simulink model "attitude_kalman_filter"  (R2023a)
settings: configuration reference "configuration_filter" (kept outside this file)
undefined symbols (not defined in the file): correction_performed_bool, Eul_rad, filt, rot_K_est_bias_OB_B_radDs, rot_K_est_OB_B_radDs, sfor_est_B_mDs, sfor_est_bias_B_mDs2
libraries: lib_jacobians x5, lib_kinematics x1
settings Model: Creator=FC_dev1  LastModifiedBy=FC_dev1
settings ConfigSetRef: SourceName=configuration_filter  SourceLocation=Base Workspace

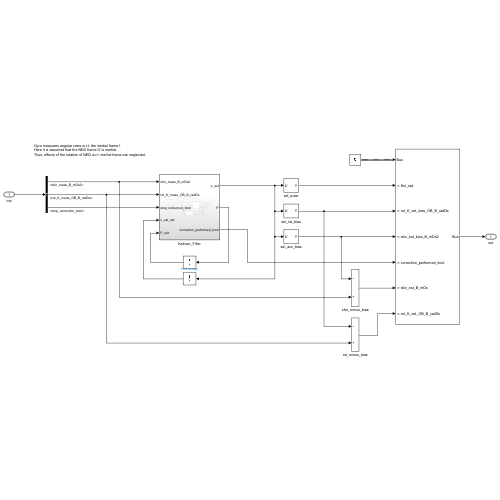
[thumbnail: Simulink's stored preview of the top-level diagram]
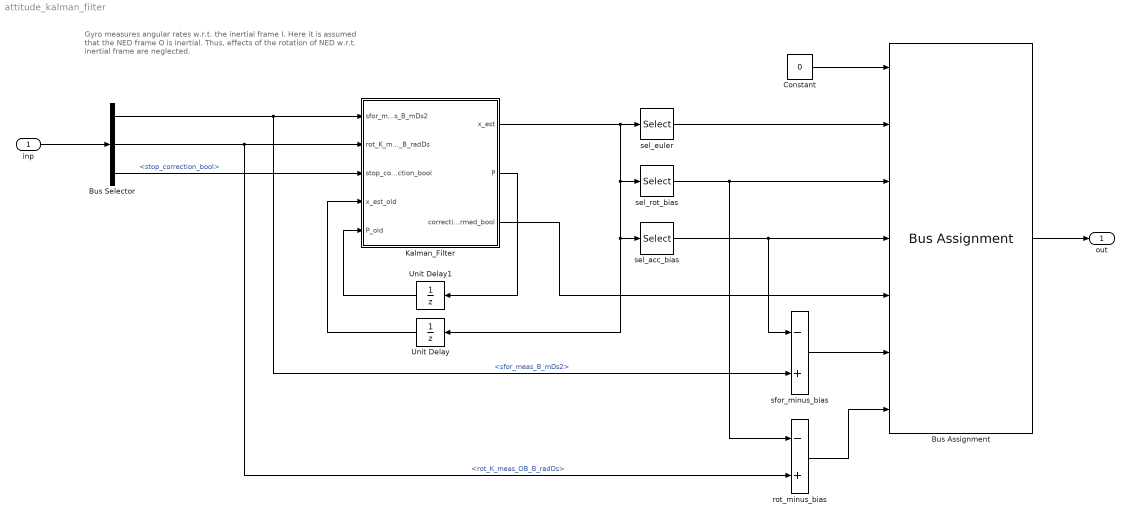
== system attitude_kalman_filter ==
  note: Gyro measures angular rates w.r.t. the inertial frame I.
      | Here it is assumed that the NED frame O is inertial.
      | Thus, effects of the rotation of NED w.r.t. inertial frame are neglected.
  inp : Inport  OutDataTypeStr=Bus: inp_Bus
  Bus Assignment : BusAssignment  AssignedSignals=Eul_rad,rot_K_est_bias_OB_B_radDs,sfor_est_bias_B_mDs2,correction_performed_bool,sfor_est_B_mDs,rot_K_est_OB_B_radDs
  Bus Selector : BusSelector  OutputSignals=sfor_meas_B_mDs2,rot_K_meas_OB_B_radDs,stop_correction_bool
  Constant : Constant  Value=0  OutDataTypeStr=Bus: out_Bus
  Kalman_Filter : Subsystem
  Unit Delay : UnitDelay  InitialCondition=filt.x0  SampleTime=-1  HasFrameUpgradeWarning=on
  Unit Delay1 : UnitDelay  InitialCondition=filt.P0  SampleTime=-1  HasFrameUpgradeWarning=on
  rot_minus_bias : Sum  Inputs=-+
  sel_acc_bias : Selector  NumberOfDimensions=2  InputPortWidth=3  IndexOptions=Index vector (dialog),Index vector (dialog)  Indices=filt.acc_bias_idx,1  OutputSizes=1,1
  sel_euler : Selector  NumberOfDimensions=2  InputPortWidth=3  IndexOptions=Index vector (dialog),Index vector (dialog)  Indices=filt.eul_idx,1  OutputSizes=1,1
  sel_rot_bias : Selector  NumberOfDimensions=2  InputPortWidth=3  IndexOptions=Index vector (dialog),Index vector (dialog)  Indices=filt.rot_bias_idx,1  OutputSizes=1,1
  sfor_minus_bias : Sum  Inputs=-+
  out : Outport  OutDataTypeStr=Bus: out_Bus
  wires:
  sel_euler/1 -> Bus Assignment/2
  Kalman_Filter/2(P) -> Unit Delay1/1
  Bus Selector/1 -> sfor_minus_bias/2, Kalman_Filter/1(sfor_meas_B_mDs2)  "<sfor_meas_B_mDs2>"
  Bus Selector/2 -> rot_minus_bias/2, Kalman_Filter/2(rot_K_meas_OB_B_radDs)  "<rot_K_meas_OB_B_radDs>"
  Unit Delay1/1 -> Kalman_Filter/5(P_old)
  Unit Delay/1 -> Kalman_Filter/4(x_est_old)
  Bus Selector/3 -> Kalman_Filter/3(stop_correction_bool)  "<stop_correction_bool>"
  Kalman_Filter/1(x_est) -> sel_rot_bias/1, Unit Delay/1, sel_acc_bias/1, sel_euler/1
  sel_rot_bias/1 -> Bus Assignment/3, rot_minus_bias/1
  sel_acc_bias/1 -> sfor_minus_bias/1, Bus Assignment/4
  Kalman_Filter/3(correction_performed_bool) -> Bus Assignment/5
  sfor_minus_bias/1 -> Bus Assignment/6
  rot_minus_bias/1 -> Bus Assignment/7
  Constant/1 -> Bus Assignment/1
  Bus Assignment/1 -> out/1
  inp/1 -> Bus Selector/1

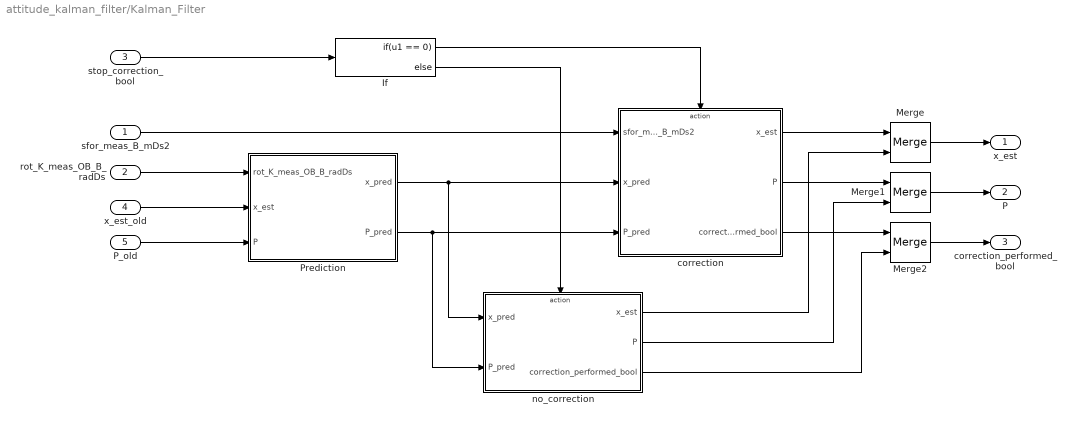
== system attitude_kalman_filter/Kalman_Filter ==
  sfor_meas_B_mDs2 : Inport
  rot_K_meas_OB_B_radDs : Inport  Port=2
  stop_correction_bool : Inport  Port=3
  x_est_old : Inport  Port=4
  P_old : Inport  Port=5
  If : If  IfExpression=u1 == 0
  Merge : Merge
  Merge1 : Merge
  Merge2 : Merge
  Prediction : Subsystem
  correction : Subsystem
  no_correction : Subsystem
  x_est : Outport
  P : Outport  Port=2
  correction_performed_bool : Outport  Port=3
  wires:
  Prediction/2(P_pred) -> correction/3(P_pred), no_correction/2(P_pred)
  x_est_old/1 -> Prediction/2(x_est)
  correction/2(P) -> Merge1/1
  sfor_meas_B_mDs2/1 -> correction/1(sfor_meas_B_mDs2)
  Prediction/1(x_pred) -> correction/2(x_pred), no_correction/1(x_pred)
  rot_K_meas_OB_B_radDs/1 -> Prediction/1(rot_K_meas_OB_B_radDs)
  correction/1(x_est) -> Merge/1
  P_old/1 -> Prediction/3(P)
  stop_correction_bool/1 -> If/1
  If/1 -> correction/Action
  Merge/1 -> x_est/1
  Merge1/1 -> P/1
  If/2 -> no_correction/Action
  no_correction/1(x_est) -> Merge/2
  no_correction/2(P) -> Merge1/2
  Merge2/1 -> correction_performed_bool/1
  correction/3(correction_performed_bool) -> Merge2/1
  no_correction/3(correction_performed_bool) -> Merge2/2

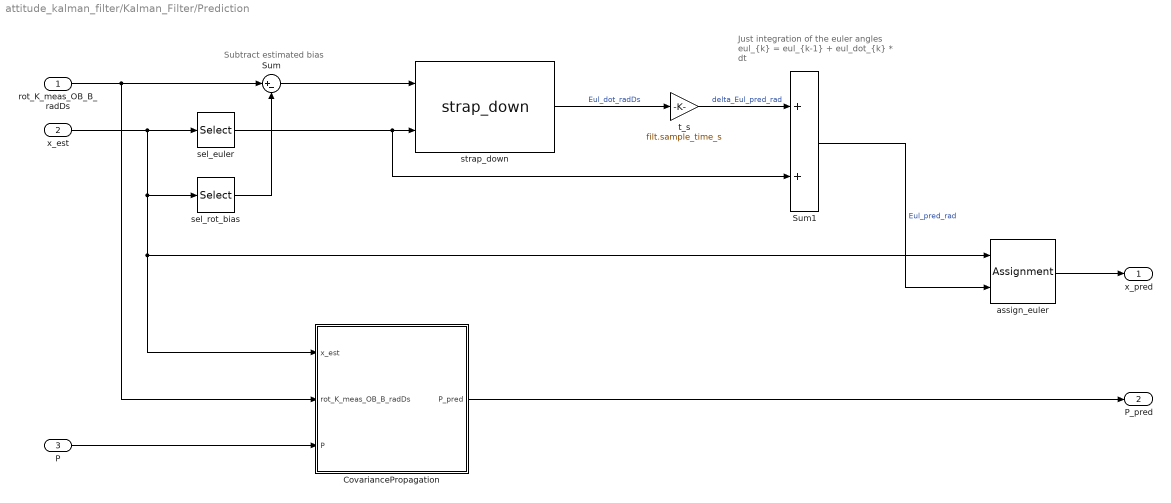
== system attitude_kalman_filter/Kalman_Filter/Prediction ==
  note: Just integration of the euler angles
      | eul_{k} = eul_{k-1} + eul_dot_{k} * dt
  note: Subtract estimated bias
  rot_K_meas_OB_B_radDs : Inport
  x_est : Inport  Port=2
  P : Inport  Port=3
  CovariancePropagation : Subsystem
  Sum : Sum  Inputs=|+-
  Sum1 : Sum
  assign_euler : Assignment  NumberOfDimensions=2  DiagnosticForDimensions=Warning  IndexOptions=Index vector (dialog),Index vector (dialog)  Indices=filt.eul_idx,1  OutputSizes=1,1
  sel_euler : Selector  NumberOfDimensions=2  InputPortWidth=3  IndexOptions=Index vector (dialog),Index vector (dialog)  Indices=filt.eul_idx,1  OutputSizes=1,1
  sel_rot_bias : Selector  NumberOfDimensions=2  InputPortWidth=3  IndexOptions=Index vector (dialog),Index vector (dialog)  Indices=filt.rot_bias_idx,1  OutputSizes=1,1
  strap_down : lib_kinematics/strap_down  SystemSampleTime=-1  VariantActivationTime=update diagram  Latency=0  AutoFrameSizeCalculation=off
  t_s : Gain  Gain=filt.sample_time_s
  x_pred : Outport
  P_pred : Outport  Port=2
  wires:
  rot_K_meas_OB_B_radDs/1 -> CovariancePropagation/2(rot_K_meas_OB_B_radDs), Sum/1
  x_est/1 -> CovariancePropagation/1(x_est), assign_euler/1, sel_rot_bias/1, sel_euler/1
  P/1 -> CovariancePropagation/3(P)
  CovariancePropagation/1(P_pred) -> P_pred/1
  sel_euler/1 -> Sum1/2, strap_down/2
  Sum/1 -> strap_down/1
  sel_rot_bias/1 -> Sum/2
  strap_down/1 -> t_s/1  "Eul_dot_radDs"
  t_s/1 -> Sum1/1  "delta_Eul_pred_rad"
  Sum1/1 -> assign_euler/2  "Eul_pred_rad"
  assign_euler/1 -> x_pred/1

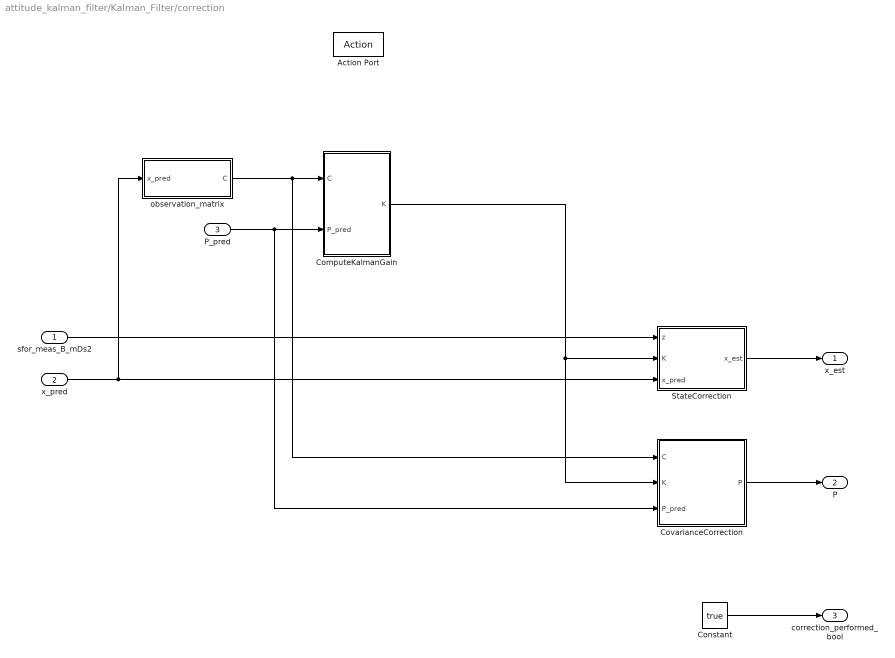
== system attitude_kalman_filter/Kalman_Filter/correction ==
  sfor_meas_B_mDs2 : Inport
  x_pred : Inport  Port=2
  P_pred : Inport  Port=3
  Action Port : ActionPort  ActionPortLabel=if(u1 == 0)
  ComputeKalmanGain : Subsystem
  Constant : Constant  Value=true
  CovarianceCorrection : Subsystem
  StateCorrection : Subsystem
  observation_matrix : Subsystem
  x_est : Outport
  P : Outport  Port=2
  correction_performed_bool : Outport  Port=3
  wires:
  P_pred/1 -> CovarianceCorrection/3(P_pred), ComputeKalmanGain/2(P_pred)
  observation_matrix/1(C) -> CovarianceCorrection/1(C), ComputeKalmanGain/1(C)
  StateCorrection/1(x_est) -> x_est/1
  CovarianceCorrection/1(P) -> P/1
  x_pred/1 -> observation_matrix/1(x_pred), StateCorrection/3(x_pred)
  ComputeKalmanGain/1(K) -> CovarianceCorrection/2(K), StateCorrection/2(K)
  sfor_meas_B_mDs2/1 -> StateCorrection/1(z)
  Constant/1 -> correction_performed_bool/1

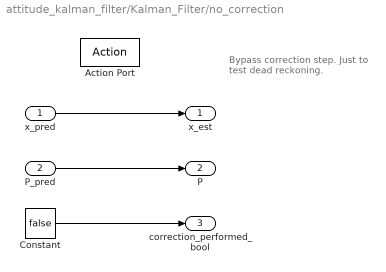
== system attitude_kalman_filter/Kalman_Filter/no_correction ==
  note: Bypass correction step.
      | Just to test dead reckoning.
  x_pred : Inport
  P_pred : Inport  Port=2
  Action Port : ActionPort  ActionPortLabel=else
  Constant : Constant  Value=false
  x_est : Outport
  P : Outport  Port=2
  correction_performed_bool : Outport  Port=3
  wires:
  P_pred/1 -> P/1
  x_pred/1 -> x_est/1
  Constant/1 -> correction_performed_bool/1

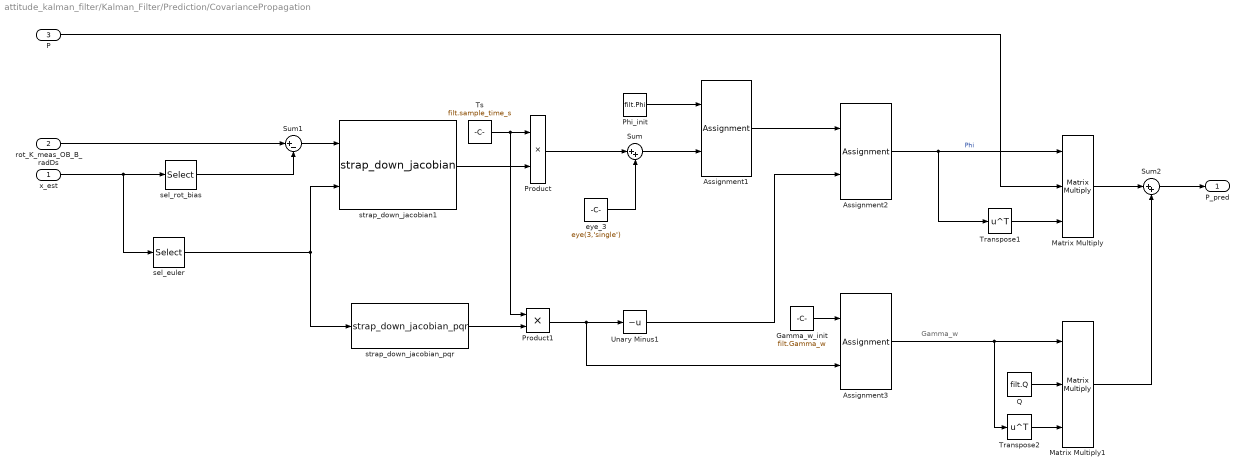
== system attitude_kalman_filter/Kalman_Filter/Prediction/CovariancePropagation ==
  note: Gamma_w
  x_est : Inport
  rot_K_meas_OB_B_radDs : Inport  Port=2
  P : Inport  Port=3
  Assignment1 : Assignment  NumberOfDimensions=2  DiagnosticForDimensions=Warning  IndexOptions=Index vector (dialog),Index vector (dialog)  Indices=filt.eul_idx,filt.eul_idx  OutputSizes=1,1
  Assignment2 : Assignment  NumberOfDimensions=2  DiagnosticForDimensions=Warning  IndexOptions=Index vector (dialog),Index vector (dialog)  Indices=filt.rot_bias_idx,filt.rot_bias_idx  OutputSizes=1,1
  Assignment3 : Assignment  NumberOfDimensions=2  DiagnosticForDimensions=Warning  IndexOptions=Index vector (dialog),Index vector (dialog)  Indices=filt.eul_idx,filt.rot_noise_idx  OutputSizes=1,1
  Gamma_w_init : Constant  Value=filt.Gamma_w  VectorParams1D=off
  Matrix Multiply : Product  Inputs=3  Multiplication=Matrix(*)
  Matrix Multiply1 : Product  Inputs=3  Multiplication=Matrix(*)
  Phi_init : Constant  Value=filt.Phi  VectorParams1D=off
  Product : Product
  Product1 : Product
  Q : Constant  Value=filt.Q  VectorParams1D=off
  Sum : Sum  Inputs=|++
  Sum1 : Sum  Inputs=|+-
  Sum2 : Sum  Inputs=|++
  Transpose1 : Math  Operator=transpose
  Transpose2 : Math  Operator=transpose
  Ts : Constant  Value=filt.sample_time_s
  Unary Minus1 : UnaryMinus
  eye_3 : Constant  Value=eye(3,'single')  VectorParams1D=off
  sel_euler : Selector  NumberOfDimensions=2  InputPortWidth=3  IndexOptions=Index vector (dialog),Index vector (dialog)  Indices=filt.eul_idx,1  OutputSizes=1,1
  sel_rot_bias : Selector  NumberOfDimensions=2  InputPortWidth=3  IndexOptions=Index vector (dialog),Index vector (dialog)  Indices=filt.rot_bias_idx,1  OutputSizes=1,1
  strap_down_jacobian1 : lib_jacobians/strap_down_jacobian  SystemSampleTime=-1  VariantActivationTime=update diagram  Latency=0  AutoFrameSizeCalculation=off
  strap_down_jacobian_pqr : lib_jacobians/strap_down_jacobian_pqr  SystemSampleTime=-1  VariantActivationTime=update diagram  Latency=0  AutoFrameSizeCalculation=off
  P_pred : Outport
  wires:
  P/1 -> Matrix Multiply/2
  Transpose1/1 -> Matrix Multiply/3
  x_est/1 -> sel_rot_bias/1, sel_euler/1
  sel_euler/1 -> strap_down_jacobian1/2, strap_down_jacobian_pqr/1
  rot_K_meas_OB_B_radDs/1 -> Sum1/1
  sel_rot_bias/1 -> Sum1/2
  strap_down_jacobian1/1 -> Product/2
  Product/1 -> Sum/1
  Phi_init/1 -> Assignment1/1
  Sum/1 -> Assignment1/2
  eye_3/1 -> Sum/2
  strap_down_jacobian_pqr/1 -> Product1/2
  Sum1/1 -> strap_down_jacobian1/1
  Product1/1 -> Unary Minus1/1, Assignment3/2
  Assignment1/1 -> Assignment2/1
  Unary Minus1/1 -> Assignment2/2
  Gamma_w_init/1 -> Assignment3/1
  Assignment2/1 -> Matrix Multiply/1, Transpose1/1  "Phi"
  Assignment3/1 -> Transpose2/1, Matrix Multiply1/1
  Transpose2/1 -> Matrix Multiply1/3
  Q/1 -> Matrix Multiply1/2
  Matrix Multiply/1 -> Sum2/1
  Sum2/1 -> P_pred/1
  Matrix Multiply1/1 -> Sum2/2
  Ts/1 -> Product1/1, Product/1

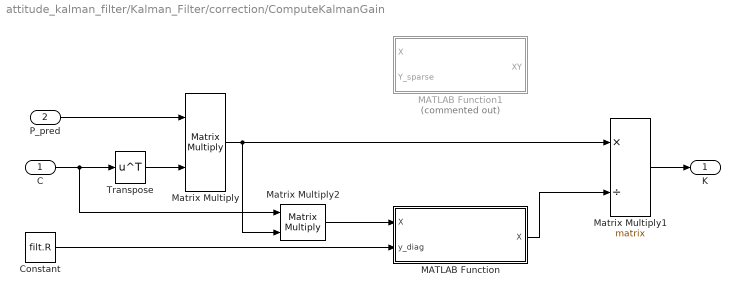
== system attitude_kalman_filter/Kalman_Filter/correction/ComputeKalmanGain ==
  C : Inport
  P_pred : Inport  Port=2
  Constant : Constant  Value=filt.R
  MATLAB Function : MATLAB Function  TreatAsAtomicUnit=on
  MATLAB Function1 : MATLAB Function  Commented=on  TreatAsAtomicUnit=on
  Matrix Multiply : Product  Multiplication=Matrix(*)
  Matrix Multiply1 : Product  Inputs=*/  Multiplication=Matrix(*)
  Matrix Multiply2 : Product  Multiplication=Matrix(*)
  Transpose : Math  Operator=transpose
  K : Outport
  wires:
  P_pred/1 -> Matrix Multiply/1
  Matrix Multiply/1 -> Matrix Multiply1/1, Matrix Multiply2/2
  C/1 -> Matrix Multiply2/1, Transpose/1
  Transpose/1 -> Matrix Multiply/2
  Matrix Multiply2/1 -> MATLAB Function/1("X ")
  MATLAB Function/1(X) -> Matrix Multiply1/2
  Constant/1 -> MATLAB Function/2(y_diag)
  Matrix Multiply1/1 -> K/1

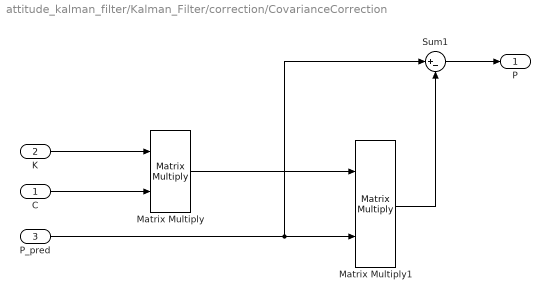
== system attitude_kalman_filter/Kalman_Filter/correction/CovarianceCorrection ==
  C : Inport
  K : Inport  Port=2
  P_pred : Inport  Port=3
  Matrix Multiply : Product  Multiplication=Matrix(*)
  Matrix Multiply1 : Product  Multiplication=Matrix(*)
  Sum1 : Sum  Inputs=|+-
  P : Outport
  wires:
  C/1 -> Matrix Multiply/2
  K/1 -> Matrix Multiply/1
  Matrix Multiply/1 -> Matrix Multiply1/1
  Matrix Multiply1/1 -> Sum1/2
  P_pred/1 -> Sum1/1, Matrix Multiply1/2
  Sum1/1 -> P/1

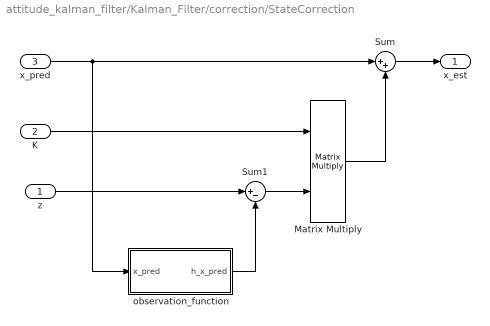
== system attitude_kalman_filter/Kalman_Filter/correction/StateCorrection ==
  z : Inport
  K : Inport  Port=2
  x_pred : Inport  Port=3
  Matrix Multiply : Product  Multiplication=Matrix(*)
  Sum : Sum  Inputs=|++
  Sum1 : Sum  Inputs=|+-
  observation_function : Subsystem
  x_est : Outport
  wires:
  x_pred/1 -> observation_function/1(x_pred), Sum/1
  K/1 -> Matrix Multiply/1
  Matrix Multiply/1 -> Sum/2
  Sum/1 -> x_est/1
  z/1 -> Sum1/1
  observation_function/1(h_x_pred) -> Sum1/2
  Sum1/1 -> Matrix Multiply/2

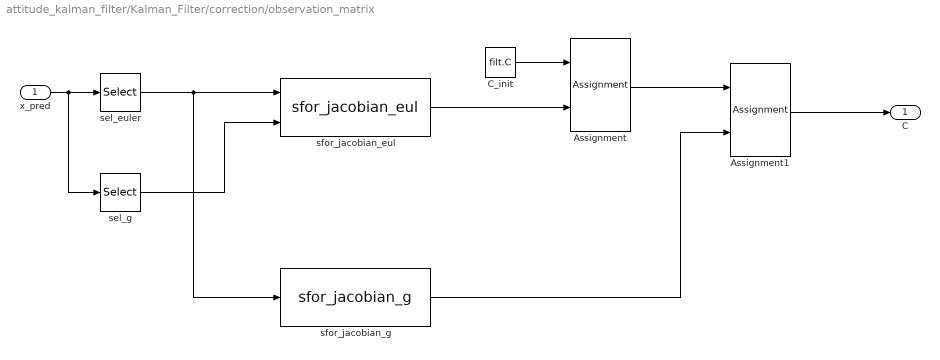
== system attitude_kalman_filter/Kalman_Filter/correction/observation_matrix ==
  x_pred : Inport
  Assignment : Assignment  NumberOfDimensions=2  DiagnosticForDimensions=Warning  IndexOptions=Assign all,Index vector (dialog)  Indices=1,filt.eul_idx  OutputSizes=1,1
  Assignment1 : Assignment  NumberOfDimensions=2  DiagnosticForDimensions=Warning  IndexOptions=Assign all,Index vector (dialog)  Indices=1,filt.g_idx  OutputSizes=1,1
  C_init : Constant  Value=filt.C  VectorParams1D=off
  sel_euler : Selector  NumberOfDimensions=2  InputPortWidth=3  IndexOptions=Index vector (dialog),Index vector (dialog)  Indices=filt.eul_idx,1  OutputSizes=1,1
  sel_g : Selector  NumberOfDimensions=2  InputPortWidth=3  IndexOptions=Index vector (dialog),Index vector (dialog)  Indices=filt.g_idx,1  OutputSizes=1,1
  sfor_jacobian_eul : lib_jacobians/sfor_jacobian_eul  SystemSampleTime=-1  VariantActivationTime=update diagram  Latency=0  AutoFrameSizeCalculation=off
  sfor_jacobian_g : lib_jacobians/sfor_jacobian_g  SystemSampleTime=-1  VariantActivationTime=update diagram  Latency=0  AutoFrameSizeCalculation=off
  C : Outport
  wires:
  x_pred/1 -> sel_g/1, sel_euler/1
  sel_euler/1 -> sfor_jacobian_eul/1, sfor_jacobian_g/1
  sel_g/1 -> sfor_jacobian_eul/2
  C_init/1 -> Assignment/1
  sfor_jacobian_eul/1 -> Assignment/2
  Assignment/1 -> Assignment1/1
  Assignment1/1 -> C/1
  sfor_jacobian_g/1 -> Assignment1/2

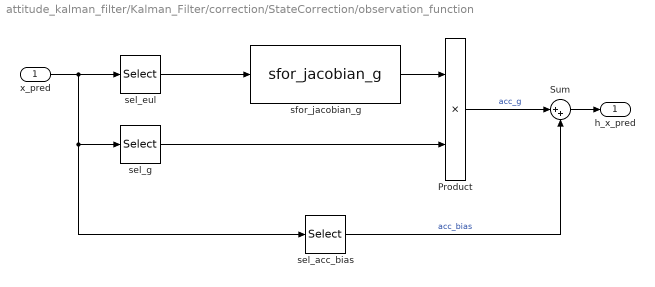
== system attitude_kalman_filter/Kalman_Filter/correction/StateCorrection/observation_function ==
  x_pred : Inport
  Product : Product
  Sum : Sum  Inputs=|++
  sel_acc_bias : Selector  NumberOfDimensions=2  InputPortWidth=3  IndexOptions=Index vector (dialog),Index vector (dialog)  Indices=filt.acc_bias_idx,1  OutputSizes=1,1
  sel_eul : Selector  NumberOfDimensions=2  InputPortWidth=3  IndexOptions=Index vector (dialog),Index vector (dialog)  Indices=filt.eul_idx,1  OutputSizes=1,1
  sel_g : Selector  NumberOfDimensions=2  InputPortWidth=3  IndexOptions=Index vector (dialog),Index vector (dialog)  Indices=filt.g_idx,1  OutputSizes=1,1
  sfor_jacobian_g : lib_jacobians/sfor_jacobian_g  SystemSampleTime=-1  VariantActivationTime=update diagram  Latency=0  AutoFrameSizeCalculation=off
  h_x_pred : Outport
  wires:
  x_pred/1 -> sel_acc_bias/1, sel_g/1, sel_eul/1
  Sum/1 -> h_x_pred/1
  sel_acc_bias/1 -> Sum/2  "acc_bias"
  sel_eul/1 -> sfor_jacobian_g/1
  sfor_jacobian_g/1 -> Product/1
  sel_g/1 -> Product/2
  Product/1 -> Sum/1  "acc_g"

== matlab function attitude_kalman_filter/Kalman_Filter/correction/ComputeKalmanGain/MATLAB Function1 ==
  data: X input; XY output; Y_sparse input
function XY = matrix_multiply(X, Y_sparse)

l = length(X(:,1));
m = length(Y_sparse(1,:));

XY = zeros(l,m,'single');

for ii = 1:N
    
    X(ii,ii) = X(ii,ii) + y_diag(ii);

end

X = inv(X);

== matlab function attitude_kalman_filter/Kalman_Filter/correction/ComputeKalmanGain/MATLAB Function ==
  data: X input; X output; y_diag input
function X = add_diagonal(X, y_diag)

N = length(y_diag);

for ii = 1:N
    
    X(ii,ii) = X(ii,ii) + y_diag(ii);

end

X = inv(X);
